simulink model "ex4_9"  (R2020b)
settings: Solver=VariableStepAuto  StartTime=0.0  StopTime=4.096  RelTol=1e-3
libraries: dspsrcs4 x3, dsparch4 x1
settings Model: Creator=seojoon  LastModifiedBy=seojoon

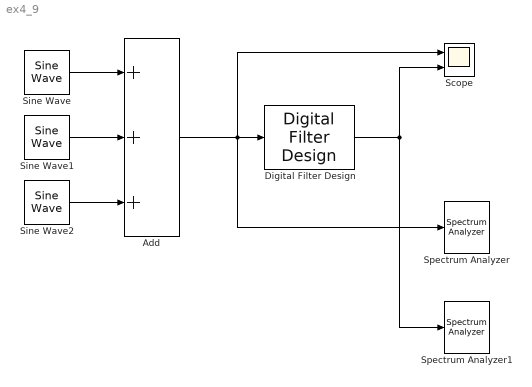
== system ex4_9 ==
  Add : Sum  Inputs=+++
  Digital Filter Design : dsparch4/Digital Filter Design  mwdsp_browser_bugfix_var=off
  Scope : Scope  NumInputPorts=2
  Sine Wave : dspsrcs4/Sine Wave  Amplitude=10  Frequency=50  Phase=0  SampleMode=Discrete  OutComplex=Real  CompMethod=Trigonometric fcn  TableSize=Speed  SampleTime=1e-3  SamplesPerFrame=1  ResetState=Restart at time zero  OutputFrames=off  dataType=double  wordLen=16  udDataType=sfix(16)  fracBitsMode=Best precision  numFracBits=15  OutDataTypeStr=double  LastOutDataTypeStr=double
  Sine Wave1 : dspsrcs4/Sine Wave  Amplitude=10  Frequency=100  Phase=pi/2  SampleMode=Discrete  OutComplex=Real  CompMethod=Trigonometric fcn  TableSize=Speed  SampleTime=1e-3  SamplesPerFrame=1  ResetState=Restart at time zero  OutputFrames=off  dataType=double  wordLen=16  udDataType=sfix(16)  fracBitsMode=Best precision  numFracBits=15  OutDataTypeStr=double  LastOutDataTypeStr=double
  Sine Wave2 : dspsrcs4/Sine Wave  Amplitude=-10  Frequency=200  Phase=pi  SampleMode=Discrete  OutComplex=Real  CompMethod=Trigonometric fcn  TableSize=Speed  SampleTime=1e-3  SamplesPerFrame=1  ResetState=Restart at time zero  OutputFrames=off  dataType=double  wordLen=16  udDataType=sfix(16)  fracBitsMode=Best precision  numFracBits=15  OutDataTypeStr=double  LastOutDataTypeStr=double
  Spectrum Analyzer : SpectrumAnalyzer
  Spectrum Analyzer1 : SpectrumAnalyzer
  wires:
  Sine Wave1/1 -> Add/2
  Add/1 -> Digital Filter Design/1, Spectrum Analyzer/1, Scope/1
  Sine Wave2/1 -> Add/3
  Sine Wave/1 -> Add/1
  Digital Filter Design/1 -> Spectrum Analyzer1/1, Scope/2
